simulink model "d"  (R2012b)
settings: Solver=ode45  StartTime=0.0  StopTime=200  RelTol=1e-3
libraries: simulink x3
settings Model: Creator=ZhouHaoyu  LastModifiedBy=ZhouHaoyu
settings DataIOCC: ExternalInput=[t,Alt,Vel]  LoadExternalInput=on

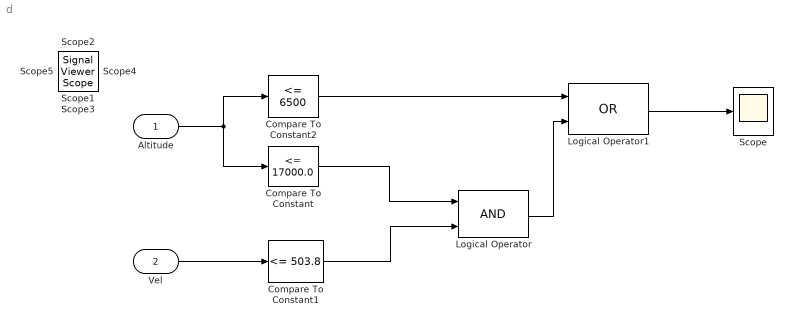
== system d ==
  Altitude : Inport
  Vel : Inport  Port=2
  Compare To Constant : simulink/Logic and Bit Operations/Compare To Constant  relop=<=  const=17000.0  OutDataTypeStr=boolean
  Compare To Constant1 : simulink/Logic and Bit Operations/Compare To Constant  relop=<=  const=503.8  OutDataTypeStr=boolean
  Compare To Constant2 : simulink/Logic and Bit Operations/Compare To Constant  relop=<=  const=6500  OutDataTypeStr=boolean
  Logical Operator : Logic  AllPortsSameDT=off  OutDataTypeStr=boolean
  Logical Operator1 : Logic  Operator=OR  AllPortsSameDT=off  OutDataTypeStr=boolean
  Scope : Scope
  Scope{1..5} (5 alike) : SignalViewerScope  IOType=viewer  RefreshTime=0.035000
      Scope3 settings: SaveName=ScopeData2
      Scope4 settings: SaveName=ScopeData3
      Scope5 settings: SaveName=ScopeData4
  wires:
  Altitude/1 -> Compare To Constant/1, Compare To Constant2/1
  Vel/1 -> Compare To Constant1/1
  Compare To Constant/1 -> Logical Operator/1
  Compare To Constant1/1 -> Logical Operator/2
  Compare To Constant2/1 -> Logical Operator1/1
  Logical Operator/1 -> Logical Operator1/2
  Logical Operator1/1 -> Scope/1
